simulink model "DSBAMDemodulator"  (R2020b)
settings: Solver=VariableStepAuto  StartTime=0.0  StopTime=2  RelTol=1e-3
libraries: dsparch4 x1
settings Model: PacingRate=0.011000  Creator=DAM  LastModifiedBy=DAM
settings SolverCC: AutoInsertRateTranBlk=on

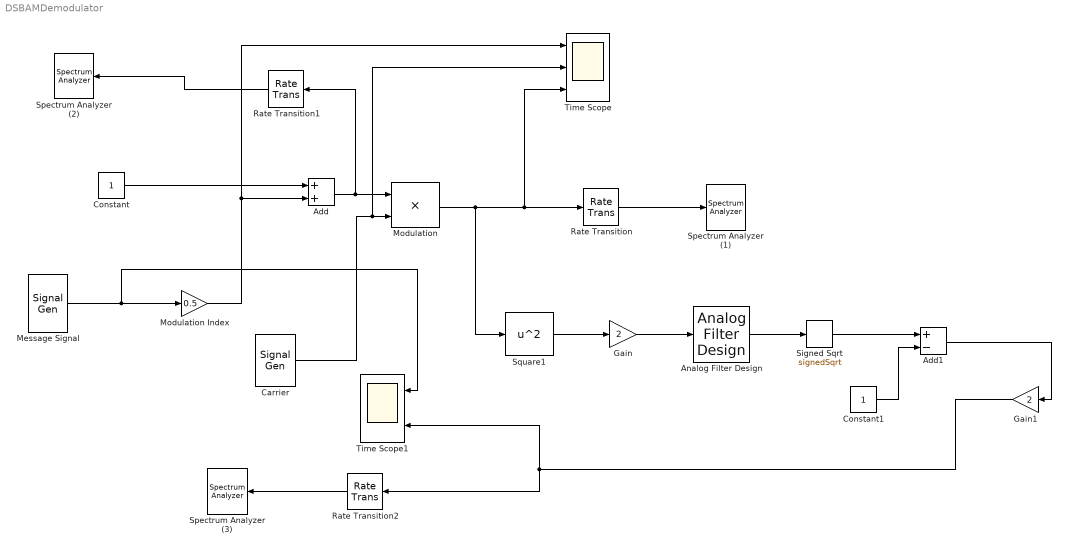
== system DSBAMDemodulator ==
  Add : Sum
  Add1 : Sum  Inputs=+-
  Analog Filter Design : dsparch4/Analog Filter Design  method=Butterworth  filttype=Lowpass  N=8  Wlo=30  Whi=80  Rp=2  Rs=40
  Carrier : SignalGenerator  Frequency=20000
  Constant : Constant
  Constant1 : Constant
  Gain : Gain  Gain=2
  Gain1 : Gain  Gain=2
  Message Signal : SignalGenerator  Frequency=1000
  Modulation : Product
  "Modulation Index " : Gain  Gain=0.5
  Rate Transition : RateTransition
  Rate Transition1 : RateTransition
  Rate Transition2 : RateTransition
  Signed Sqrt : Sqrt  Operator=signedSqrt  SaturateOnIntegerOverflow=on
  Spectrum Analyzer (1) : SpectrumAnalyzer
  Spectrum Analyzer (3) : SpectrumAnalyzer
  Spectrum Analyzer (2) : SpectrumAnalyzer
  Square1 : Math  Operator=square  SaturateOnIntegerOverflow=on
  Time Scope : Scope  NumInputPorts=3
  Time Scope1 : Scope  NumInputPorts=2
  wires:
  Add/1 -> Modulation/1, Rate Transition1/1
  Rate Transition1/1 -> Spectrum Analyzer (2)/1
  "Modulation Index "/1 -> Time Scope/1, Add/2
  Constant/1 -> Add/1
  Message Signal/1 -> Time Scope1/1, "Modulation Index "/1
  Carrier/1 -> Time Scope/2, Modulation/2
  Modulation/1 -> Square1/1, Time Scope/3, Rate Transition/1
  Rate Transition/1 -> Spectrum Analyzer (1)/1
  Square1/1 -> Gain/1
  Gain/1 -> Analog Filter Design/1
  Analog Filter Design/1 -> Signed Sqrt/1
  Signed Sqrt/1 -> Add1/1
  Constant1/1 -> Add1/2
  Add1/1 -> Gain1/1
  Gain1/1 -> Time Scope1/2, Rate Transition2/1
  Rate Transition2/1 -> Spectrum Analyzer (3)/1
